simulink model "HydrogenRefuelingStation_Param"  (R2023b)
settings: Solver=VariableStepAuto  StartTime=0.0  StopTime=finSimulation  RelTol=1e-3  AbsTol=1e-3
PreLoadFcn:
  | load hydrogen_properties.mat
  | load silicone_fluid_properties.mat
  | 
  | p_storage = 200; % [bar]
  | p_vehicle_init = 100; % [bar]
  | T_env = 25; % [degC]
  | T_fluid = -60; % [degC]
  | 
  | V_vehicle = 172; % [l]
  | 
  | tube_D = 0.04; % [m]
  | hose_D = 0.0064; % [m]
  | pipe_D = 0.1; % [m]
  | 
  | num_buffer = 2;
  | 
  | intercooler_num_tubes = 25;
  | intercooler_tube_D = 0.008; % [m]
  | intercooler_shell_D = 0.1; % [m]
  | intercooler_L = 2; % [m]
  | 
  | precooler_tube_W = 0.001; % [m]
  | precooler_num_tubes = 50*25;
  | precooler_L = 1; % [m]
values from neighbouring files (symbols this model uses):
  EngDemandTime = 3000    [launch.m]
  EngThrottle = 1    [launch.m]
  ext_bufferEng_D = 0.025    [System_Parameters.m]
  ext_Manifold_D = 0.007    [System_Parameters.m]
  ext_vehTank_D = 0.25    [System_Parameters.m]
  in_bufferEng_D = 0.0064    [System_Parameters.m]
  in_Eng_D = 0.0064    [System_Parameters.m]
  in_Man_D = 0.0064    [System_Parameters.m]
  inOut_vehTank_D = 0.0064    [System_Parameters.m]
  int_bufferEng_D = 0.024    [System_Parameters.m]
  int_Manifold_D = 0.0064    [System_Parameters.m]
  int_vehTank_D = 0.22    [System_Parameters.m]
  L_bufferEng = 1    [System_Parameters.m]
  L_Manifold = 1    [System_Parameters.m]
  L_vehTank = 2    [System_Parameters.m]
  MV_D = 0.0064    [System_Parameters.m]
  out_bufferEng_D = 0.0064/2    (= 0.0032)    [System_Parameters.m]
  out_Eng_D = 0.0064    [System_Parameters.m]
  out_Man_D = 0.0064    [System_Parameters.m]
  Pipe_ConnMan_D = 0.0064    [System_Parameters.m]
  Pipe_ManPR_D = 0.0064    [System_Parameters.m]
  Pipe_ManTank_D = 0.0064    [System_Parameters.m]
  Pipe_PRBuffer_D = 0.0064    [System_Parameters.m]
  redn_PR_D = 0.0064    [System_Parameters.m]
  redn_PR_setP = 160    [System_Parameters.m]
  relief_PR_D = 0.0064    [System_Parameters.m]
  relief_vehTank_D = 0.0064    [System_Parameters.m]
  silicone_fluid =     [silicone_fluid_properties.mat]
  statConn_D = 0.0064    [System_Parameters.m]
  stationTrigger_Time = 2400    [System_Parameters.m]
  SV_D = 0.0064    [System_Parameters.m]
  tank_Man_D = 0.0064    [System_Parameters.m]
  TempCont_vehTank_D = 0.0064    [System_Parameters.m]
  vehConn_D = 0.0064    [System_Parameters.m]
  WP_high = 700    [System_Parameters.m]
libraries: fl_lib x128, nesl_utility x60, SimscapeFluids_lib x41, slpidlib x4
(part 6 of 6)

== system HydrogenRefuelingStation_Param/STATION/Multistage Compressor/Stage 2 ==
  Diaphragm Compressor : SimscapeFluids_lib/Gas/Turbomachinery/Positive-Displacement Compressor (G)  dispSpec=fluids.gas.turbomachinery.enum.DisplacementSpecification.Displacement  v_disp=230 cm^3/rev  mdot_nom=0.01 kg/s  omega_nom=1000 rpm  efficiencySpec=fluids.gas.turbomachinery.enum.VolumetricEfficiencyParameterization.Analytical  thermodynamicModelSpec=fluids.gas.turbomachinery.enum.ThermodynamicModel.Polytropic  n=1.4  eta_isen=0.65  eta_isen_TLU=[.95, .9, .85, .8, .75; .925, .875, .825, .775, .725; .875, .825, .775, .725, .675; .75, .7, .65, .6, .55]  eta_vol_nom=0.9  pr_TLU=[2, 4, 6, 8]  omega_TLU=[800, 1500, 2800, 3300, 4000] rpm  eta_vol_TLU=[.95, .9, .85, .8, .75; .925, .875, .825, .775, .725; .875, .825, .775, .725, .675; .75, .7, .65, .6, .55]  pr_nom=1.8  p_in_nom=0.101325 MPa  T_in_nom=293.15 K  mechanical_efficiency=0.95  area_A=pi*tube_D^2/4 m^2  area_B=pi*tube_D^2/4 m^2
      settings: InternalSimscapePortConfiguration="{\"Bottom\":[],\"Left\":[{\"id\":\"A\",\"label\":\"A\",\"type\":\"foundation.gas.gas\"},{\"id\":\"C\",\"label\":\"C\",\"type\":\"foundation.mechanical.rotational.rotational\"}],\"Right\":[{\"id\":\"B\",\"label\":\"B\",\"type\":\"foundation.gas.gas\"},{\"id\":\"R\",\"label\":\"R\",\"type\":\"foundation.mechanical.rotational.rotational\"}],\"Top\":[]}"
  Intercooler : SimscapeFluids_lib/Fluid Network Interfaces/Heat Exchangers/Heat Exchanger (G-TL)  hex_type=fluids.interfaces.enum.flow_arrangement_spec.parallel_counter  shell_num=1  cross_type=fluids.interfaces.enum.cross_flow_heat_exchanger_G_TL_spec.mixed_mixed  NTU_TLU=[.5, 1, 2, 3, 4, 5]  CR_TLU=[0, .25, .5, .75, 1]  eff_TLU=[.3, .3, .3, .3, .3; .6, .55, .5, .47, .43; .85, .76, .68, .61, .55; .94, .83, .72, .65, .58; .98, .86, .75, .66, .58; .99, .86, .75, .66, .58]  wall_thermal_dynamics=simscape.enum.onoff.off  thermal_mass_wall=447 J/K  R_wall=0 K/W  min_flow_area_1=intercooler_num_tubes * pi * intercooler_tube_D^2 / 4 m^2  Dh_press_1=intercooler_tube_D m  gas_volume_1=intercooler_num_tubes * pi * intercooler_tube_D^2 / 4 * intercooler_L m^3  Re_lam_1=2000  Re_tur_1=4000  pressure_loss_spec_1=fluids.interfaces.enum.pressure_loss_spec.tube_correlation  pressure_loss_coeff_1=0.1  length_press_1=intercooler_L m  length_add_1=0.3 m  roughness_1=15e-6 m  Re_friction_TLU_1=[400, 1000, 1500, 3000, 4000, 6000, 10000, 20000, 40000, 60000, 100000, 100000000]  friction_factor_TLU_1=[.264, .112, .071, .0417, .0387, .0268, .025, .0232, .0226, .022, .0214, .0214]  shape_factor_1=64  Re_Euler_TLU_1=[50, 500, 1000, 2000]  Euler_TLU_1=[4.4505, .6864, .4791, .3755]  heat_transfer_spec_1=fluids.interfaces.enum.heat_transfer_spec.tube_correlation  heat_transfer_area_1=intercooler_num_tubes * pi * intercooler_tube_D * intercooler_L m^2  heat_coeff_1=100 W/(K*m^2)  length_heat_1=intercooler_L m  Nu_lam_1=3.66  Re_Colburn_TLU_1=[100, 150, 1000]  Colburn_factor_TLU_1=[.019, .013, .002]  Re_Nu_TLU_1=[100, 150, 1000]  Pr_Nu_TLU_1=[1, 10]  Nu_TLU_1=[3.72, 4.21; 3.75, 4.44; 4.21, 7.15]  fouling_factor_1=0 K*m^2/W  mdot_threshold_1=1e-6 kg/s  min_heat_coeff_1=5 W/(K*m^2)  min_flow_area_2=pi * (intercooler_shell_D^2 - intercooler_num_tubes * intercooler_tube_D^2) / 4 m^2  Dh_press_2=|  liquid_volume_2=pi * (intercooler_shell_D^2 - intercooler_num_tubes * intercooler_tube_D^2) / 4 * intercooler_L m^3  Re_lam_2=2000  Re_tur_2=4000  pressure_loss_spec_2=fluids.interfaces.enum.pressure_loss_spec.tube_correlation  pressure_loss_coeff_2=0.1  length_press_2=intercooler_L m  length_add_2=0.3 m  roughness_2=15e-6 m  Re_friction_TLU_2=[400, 1000, 1500, 3000, 4000, 6000, 10000, 20000, 40000, 60000, 100000, 100000000]  friction_factor_TLU_2=[.264, .112, .071, .0417, .0387, .0268, .025, .0232, .0226, .022, .0214, .0214]  shape_factor_2=64  Re_Euler_TLU_2=[50, 500, 1000, 2000]  Euler_TLU_2=[4.4505, .6864, .4791, .3755]  heat_transfer_spec_2=fluids.interfaces.enum.heat_transfer_spec.tube_correlation  heat_transfer_area_2=intercooler_num_tubes * pi * intercooler_tube_D * intercooler_L m^2  heat_coeff_2=100 W/(K*m^2)  length_heat_2=intercooler_L m  Nu_lam_2=3.66  Re_Colburn_TLU_2=[100, 150, 1000]  Colburn_factor_TLU_2=[.019, .013, .002]  Re_Nu_TLU_2=[100, 150, 1000]  Pr_Nu_TLU_2=[1, 10]  Nu_TLU_2=[3.72, 4.21; 3.75, 4.44; 4.21, 7.15]  fouling_factor_2=0 K*m^2/W  min_heat_coeff_2=5 W/(K*m^2)  T0_1=T_env degC  p0_1=p_storage bar  dynamic_compressibility_2=simscape.enum.onoff.on  T0_2=T_env degC  p0_2=0.101325 MPa  mdot1_TLU=[.3, .5, .6, .7, 1, 1.4, 1.9, 2.3] kg/s  mdot2_TLU=[.3, .5, 1, 1.3, 1.7, 2, 2.6, 3.3] kg/s  SD_TLU=[.324, .3533, .404, .4253, .4333, .4373, .4453, .4533; .3813, .424, .496, .5307, .544, .5547, .5693, .5787; .4267, .4827, .5813, .6173, .6413, .6573, .672, .6827; .4613, .528, .64, .6987, .7267, .7467, .7707, .7853; .5533, .6467, .8227, .928, .9853, 1.0187, 1.0653, 1.0973; .58, .688, .8853, 1.0147, 1.08, 1.124, 1.176, 1.2147; .624, .7467, .992, 1.148, 1.244, 1.304, 1.3773, 1.4267; .656, .7907, 1.0667, 1.26, 1.376, 1.452, 1.548, 1.612] kW/K  Q_check=fluids.interfaces.enum.SD_max_check.warning  mdot_dp_TLU_1=[.3, .5, 1, 1.5, 2, 2.5] kg/s  p_diff_TLU_1=[3, 5, 10, 25, 35, 50] * 1e-3 MPa  T_ref_in_1=293.15 K  p_ref_in_1=0.101325 MPa  area_1=0.01 m^2  mdot_dp_TLU_2=[.3, .5, 1, 1.5, 2, 2.5] kg/s  p_diff_TLU_2=[3, 5, 10, 25, 35, 50] * 1e-3 MPa  T_ref_in_2=293.15 K  p_ref_in_2=0.101325 MPa  mdot_threshold_2=1e-3 kg/s  area_2=0.01 m^2
      | (intercooler_shell_D^2 - intercooler_num_tubes * intercooler_tube_D^2) / (intercooler_shell_D + intercooler_num_tubes * intercooler_tube_D)
      |  m
      settings: InternalSimscapePortConfiguration="{\"Bottom\":[],\"Left\":[{\"id\":\"A1\",\"label\":\"A1\",\"type\":\"foundation.gas.gas\"},{\"id\":\"B1\",\"label\":\"B1\",\"type\":\"foundation.gas.gas\"}],\"Right\":[{\"id\":\"A2\",\"label\":\"A2\",\"type\":\"foundation.thermal_liquid.thermal_liquid\"},{\"id\":\"B2\",\"label\":\"B2\",\"type\":\"foundation.thermal_liquid.thermal_liquid\"}],\"Top\":[]}"
  Mechanical Rotational Reference : fl_lib/Mechanical/Rotational Elements/Mechanical Rotational Reference
  R : PMIOPort  Side=Left
  B : PMIOPort  Port=2  Side=Left
  Ac : PMIOPort  Port=3  Side=Left
  A : PMIOPort  Port=4  Side=Right
  Bc : PMIOPort  Port=5  Side=Right
  connections:
  Mechanical Rotational Reference/LConn1 -- Diaphragm Compressor/LConn2
  Ac/RConn1 -- Intercooler/RConn2
  Bc/RConn1 -- Intercooler/RConn1
  B/RConn1 -- Intercooler/LConn2
  A/RConn1 -- Diaphragm Compressor/LConn1
  Diaphragm Compressor/RConn2 -- R/RConn1
  Intercooler/LConn1 -- Diaphragm Compressor/RConn1

== system HydrogenRefuelingStation_Param/STATION/Multistage Compressor/Stage 3 ==
  Diaphragm Compressor : SimscapeFluids_lib/Gas/Turbomachinery/Positive-Displacement Compressor (G)  dispSpec=fluids.gas.turbomachinery.enum.DisplacementSpecification.Displacement  v_disp=150 cm^3/rev  mdot_nom=0.01 kg/s  omega_nom=1000 rpm  efficiencySpec=fluids.gas.turbomachinery.enum.VolumetricEfficiencyParameterization.Analytical  thermodynamicModelSpec=fluids.gas.turbomachinery.enum.ThermodynamicModel.Polytropic  n=1.4  eta_isen=0.65  eta_isen_TLU=[.95, .9, .85, .8, .75; .925, .875, .825, .775, .725; .875, .825, .775, .725, .675; .75, .7, .65, .6, .55]  eta_vol_nom=0.9  pr_TLU=[2, 4, 6, 8]  omega_TLU=[800, 1500, 2800, 3300, 4000] rpm  eta_vol_TLU=[.95, .9, .85, .8, .75; .925, .875, .825, .775, .725; .875, .825, .775, .725, .675; .75, .7, .65, .6, .55]  pr_nom=1.8  p_in_nom=0.101325 MPa  T_in_nom=293.15 K  mechanical_efficiency=0.95  area_A=pi*tube_D^2/4 m^2  area_B=pi*tube_D^2/4 m^2
      settings: InternalSimscapePortConfiguration="{\"Bottom\":[],\"Left\":[{\"id\":\"A\",\"label\":\"A\",\"type\":\"foundation.gas.gas\"},{\"id\":\"C\",\"label\":\"C\",\"type\":\"foundation.mechanical.rotational.rotational\"}],\"Right\":[{\"id\":\"B\",\"label\":\"B\",\"type\":\"foundation.gas.gas\"},{\"id\":\"R\",\"label\":\"R\",\"type\":\"foundation.mechanical.rotational.rotational\"}],\"Top\":[]}"
  Intercooler : SimscapeFluids_lib/Fluid Network Interfaces/Heat Exchangers/Heat Exchanger (G-TL)  hex_type=fluids.interfaces.enum.flow_arrangement_spec.parallel_counter  shell_num=1  cross_type=fluids.interfaces.enum.cross_flow_heat_exchanger_G_TL_spec.mixed_mixed  NTU_TLU=[.5, 1, 2, 3, 4, 5]  CR_TLU=[0, .25, .5, .75, 1]  eff_TLU=[.3, .3, .3, .3, .3; .6, .55, .5, .47, .43; .85, .76, .68, .61, .55; .94, .83, .72, .65, .58; .98, .86, .75, .66, .58; .99, .86, .75, .66, .58]  wall_thermal_dynamics=simscape.enum.onoff.off  thermal_mass_wall=447 J/K  R_wall=0 K/W  min_flow_area_1=intercooler_num_tubes * pi * intercooler_tube_D^2 / 4 m^2  Dh_press_1=intercooler_tube_D m  gas_volume_1=intercooler_num_tubes * pi * intercooler_tube_D^2 / 4 * intercooler_L m^3  Re_lam_1=2000  Re_tur_1=4000  pressure_loss_spec_1=fluids.interfaces.enum.pressure_loss_spec.tube_correlation  pressure_loss_coeff_1=0.1  length_press_1=intercooler_L m  length_add_1=0.3 m  roughness_1=15e-6 m  Re_friction_TLU_1=[400, 1000, 1500, 3000, 4000, 6000, 10000, 20000, 40000, 60000, 100000, 100000000]  friction_factor_TLU_1=[.264, .112, .071, .0417, .0387, .0268, .025, .0232, .0226, .022, .0214, .0214]  shape_factor_1=64  Re_Euler_TLU_1=[50, 500, 1000, 2000]  Euler_TLU_1=[4.4505, .6864, .4791, .3755]  heat_transfer_spec_1=fluids.interfaces.enum.heat_transfer_spec.tube_correlation  heat_transfer_area_1=intercooler_num_tubes * pi * intercooler_tube_D * intercooler_L m^2  heat_coeff_1=100 W/(K*m^2)  length_heat_1=intercooler_L m  Nu_lam_1=3.66  Re_Colburn_TLU_1=[100, 150, 1000]  Colburn_factor_TLU_1=[.019, .013, .002]  Re_Nu_TLU_1=[100, 150, 1000]  Pr_Nu_TLU_1=[1, 10]  Nu_TLU_1=[3.72, 4.21; 3.75, 4.44; 4.21, 7.15]  fouling_factor_1=0 K*m^2/W  mdot_threshold_1=1e-6 kg/s  min_heat_coeff_1=5 W/(K*m^2)  min_flow_area_2=pi * (intercooler_shell_D^2 - intercooler_num_tubes * intercooler_tube_D^2) / 4 m^2  Dh_press_2=|  liquid_volume_2=pi * (intercooler_shell_D^2 - intercooler_num_tubes * intercooler_tube_D^2) / 4 * intercooler_L m^3  Re_lam_2=2000  Re_tur_2=4000  pressure_loss_spec_2=fluids.interfaces.enum.pressure_loss_spec.tube_correlation  pressure_loss_coeff_2=0.1  length_press_2=intercooler_L m  length_add_2=0.3 m  roughness_2=15e-6 m  Re_friction_TLU_2=[400, 1000, 1500, 3000, 4000, 6000, 10000, 20000, 40000, 60000, 100000, 100000000]  friction_factor_TLU_2=[.264, .112, .071, .0417, .0387, .0268, .025, .0232, .0226, .022, .0214, .0214]  shape_factor_2=64  Re_Euler_TLU_2=[50, 500, 1000, 2000]  Euler_TLU_2=[4.4505, .6864, .4791, .3755]  heat_transfer_spec_2=fluids.interfaces.enum.heat_transfer_spec.tube_correlation  heat_transfer_area_2=intercooler_num_tubes * pi * intercooler_tube_D * intercooler_L m^2  heat_coeff_2=100 W/(K*m^2)  length_heat_2=intercooler_L m  Nu_lam_2=3.66  Re_Colburn_TLU_2=[100, 150, 1000]  Colburn_factor_TLU_2=[.019, .013, .002]  Re_Nu_TLU_2=[100, 150, 1000]  Pr_Nu_TLU_2=[1, 10]  Nu_TLU_2=[3.72, 4.21; 3.75, 4.44; 4.21, 7.15]  fouling_factor_2=0 K*m^2/W  min_heat_coeff_2=5 W/(K*m^2)  T0_1=T_env degC  p0_1=p_storage bar  dynamic_compressibility_2=simscape.enum.onoff.on  T0_2=T_env degC  p0_2=0.101325 MPa  mdot1_TLU=[.3, .5, .6, .7, 1, 1.4, 1.9, 2.3] kg/s  mdot2_TLU=[.3, .5, 1, 1.3, 1.7, 2, 2.6, 3.3] kg/s  SD_TLU=[.324, .3533, .404, .4253, .4333, .4373, .4453, .4533; .3813, .424, .496, .5307, .544, .5547, .5693, .5787; .4267, .4827, .5813, .6173, .6413, .6573, .672, .6827; .4613, .528, .64, .6987, .7267, .7467, .7707, .7853; .5533, .6467, .8227, .928, .9853, 1.0187, 1.0653, 1.0973; .58, .688, .8853, 1.0147, 1.08, 1.124, 1.176, 1.2147; .624, .7467, .992, 1.148, 1.244, 1.304, 1.3773, 1.4267; .656, .7907, 1.0667, 1.26, 1.376, 1.452, 1.548, 1.612] kW/K  Q_check=fluids.interfaces.enum.SD_max_check.warning  mdot_dp_TLU_1=[.3, .5, 1, 1.5, 2, 2.5] kg/s  p_diff_TLU_1=[3, 5, 10, 25, 35, 50] * 1e-3 MPa  T_ref_in_1=293.15 K  p_ref_in_1=0.101325 MPa  area_1=0.01 m^2  mdot_dp_TLU_2=[.3, .5, 1, 1.5, 2, 2.5] kg/s  p_diff_TLU_2=[3, 5, 10, 25, 35, 50] * 1e-3 MPa  T_ref_in_2=293.15 K  p_ref_in_2=0.101325 MPa  mdot_threshold_2=1e-3 kg/s  area_2=0.01 m^2
      | (intercooler_shell_D^2 - intercooler_num_tubes * intercooler_tube_D^2) / (intercooler_shell_D + intercooler_num_tubes * intercooler_tube_D)
      |  m
      settings: InternalSimscapePortConfiguration="{\"Bottom\":[],\"Left\":[{\"id\":\"A1\",\"label\":\"A1\",\"type\":\"foundation.gas.gas\"},{\"id\":\"B1\",\"label\":\"B1\",\"type\":\"foundation.gas.gas\"}],\"Right\":[{\"id\":\"A2\",\"label\":\"A2\",\"type\":\"foundation.thermal_liquid.thermal_liquid\"},{\"id\":\"B2\",\"label\":\"B2\",\"type\":\"foundation.thermal_liquid.thermal_liquid\"}],\"Top\":[]}"
  Mechanical Rotational Reference : fl_lib/Mechanical/Rotational Elements/Mechanical Rotational Reference
  R : PMIOPort  Side=Left
  B : PMIOPort  Port=2  Side=Left
  Ac : PMIOPort  Port=3  Side=Left
  A : PMIOPort  Port=4  Side=Right
  Bc : PMIOPort  Port=5  Side=Right
  connections:
  Mechanical Rotational Reference/LConn1 -- Diaphragm Compressor/LConn2
  Ac/RConn1 -- Intercooler/RConn2
  Bc/RConn1 -- Intercooler/RConn1
  B/RConn1 -- Intercooler/LConn2
  A/RConn1 -- Diaphragm Compressor/LConn1
  Diaphragm Compressor/RConn2 -- R/RConn1
  Intercooler/LConn1 -- Diaphragm Compressor/RConn1

== system HydrogenRefuelingStation_Param/Buffer Tank/Buffer Tank/Valve Controller1/Filter Derivative ==
  In1 : Inport
  Gain : Gain  Gain=1/tau
  Integrator : Integrator  InitialConditionSource=external
  Sum : Sum  Inputs=|+-
  x : Outport
  dx/dt : Outport  Port=2
  wires:
  In1/1 -> Sum/1, Integrator/2
  Integrator/1 -> x/1, Sum/2
  Gain/1 -> dx/dt/1, Integrator/1
  Sum/1 -> Gain/1

== stateflow chart HydrogenRefuelingStation_Param/Control Logic ==
  settings: updateMethod=CONTINUOUS
  state BufferStatus [parallel]
    settings: executionOrder=1
    state HighPressure [parallel]
      settings: executionOrder=1
      state NotFull
        entry:
        ready(1) = false;
      state Full
        entry:
        ready(1) = true;
      BufferStatus.HighPressure.NotFull -> BufferStatus.HighPressure.Full : [p_buffer(1) >= 950]
      (default) -> BufferStatus.HighPressure.NotFull
      BufferStatus.HighPressure.Full -> BufferStatus.HighPressure.NotFull : [p_buffer(1) <= 900]
    state MediumPressure [parallel]
      settings: executionOrder=2
      state NotFull
        entry:
        ready(2) = false;
      state Full
        entry:
        ready(2) = true;
      BufferStatus.MediumPressure.NotFull -> BufferStatus.MediumPressure.Full : [p_buffer(2) >= 650]
      (default) -> BufferStatus.MediumPressure.NotFull
      BufferStatus.MediumPressure.Full -> BufferStatus.MediumPressure.NotFull : [p_buffer(2) <= 600]
    state LowPressure [parallel]
      settings: executionOrder=3
      state NotFull
        entry:
        ready(3) = false;
      state Full
        entry:
        ready(3) = true;
      BufferStatus.LowPressure.NotFull -> BufferStatus.LowPressure.Full : [p_buffer(3) >= 450]
      (default) -> BufferStatus.LowPressure.NotFull
      BufferStatus.LowPressure.Full -> BufferStatus.LowPressure.NotFull : [p_buffer(3) <= 400]
  state ChargeBuffer [parallel]
    settings: executionOrder=2
    state HighPressure
      entry:
      S_buffer_in(1) = 1;
      S_comp = 1;
    state Stop
      entry:
      S_buffer_in = [0; 0; 0];
      S_comp = 0;
    state MediumPressure
      entry:
      S_buffer_in(2) = 1;
      S_comp = 1;
    state LowPressure
      entry:
      S_buffer_in(3) = 1;
      S_comp = 1;
    ChargeBuffer.HighPressure -> ChargeBuffer.Stop : [ready(1)]
    (junction 46) -> ChargeBuffer.HighPressure [order 1] : [~ready(1)]
    (default) -> ChargeBuffer.Stop
    ChargeBuffer.Stop -> (junction 46) : [after(2,sec)]
    (junction 46) -> ChargeBuffer.MediumPressure [order 2] : [~ready(2)]
    (junction 46) -> ChargeBuffer.LowPressure [order 3] : [~ready(3)]
    ChargeBuffer.LowPressure -> ChargeBuffer.Stop : [ready(3)]
    ChargeBuffer.MediumPressure -> ChargeBuffer.Stop : [ready(2)]
  state ChargeVehicle [parallel]
    settings: executionOrder=3
    state Dispense
      entry:
      S_dispense = 1;
      state HighPressure
        entry:
        S_buffer_out(1) = 1;
        APRR = APRR_target;
      state SwitchBuffer
        entry:
        S_buffer_out = [0; 0; 0];
        APRR = 0;
      state MediumPressure
        entry:
        S_buffer_out(2) = 1;
        APRR = APRR_target;
      state LowPressure
        entry:
        S_buffer_out(3) = 1;
        APRR = APRR_target;
      ChargeVehicle.Dispense.HighPressure -> SwitchBuffer : [p_buffer(1) - p_vehicle <= 50]
      (junction 82) -> ChargeVehicle.Dispense.HighPressure [order 3] : [ready(1)]
      (default) -> SwitchBuffer
      SwitchBuffer -> (junction 82) : [after(2,sec)]
      (junction 82) -> ChargeVehicle.Dispense.MediumPressure [order 2] : [ready(2) && ...
          | p_vehicle < 550]
      (junction 82) -> ChargeVehicle.Dispense.LowPressure [order 1] : [ready(3) && ...
          | p_vehicle < 350]
      ChargeVehicle.Dispense.LowPressure -> SwitchBuffer : [p_buffer(3) - p_vehicle <= 50]
      ChargeVehicle.Dispense.MediumPressure -> SwitchBuffer : [p_buffer(2) - p_vehicle <= 50]
    state Stop
      entry:
      S_buffer_out = [0; 0; 0];
      S_dispense = 0;
    state Start
      entry:
      [APRR_target, p_target] = ...
      SAE_J2601(T_env, p_vehicle);
    (default) -> ChargeVehicle.Stop
    Dispense -> ChargeVehicle.Stop : [p_vehicle >= p_target || ~trigger]
    ChargeVehicle.Stop -> Start : [trigger]
    Start -> ChargeVehicle.Stop [order 1] : [~trigger]
    Start -> Dispense [order 2] : [p_vehicle < p_target ...
        |  && any(ready)]
  state [APRR,p_target] = SAE_J2601(T_env,p_init) [function]
  data: T_env function_input double size=1; APRR function_output; p_target function_output; p_init function_input double size=1; T_env input; p_buffer input; p_vehicle input; trigger input; APRR output; S_comp output; S_dispense output; S_buffer_in output; S_buffer_out output; APRR_target local =0; p_target local =0; ready local =[false; false; false]
